simulink model "sampled_data_system"  (R2021b)
settings: Solver=ode45  StartTime=0.0  StopTime=tfinal  FixedStep=T  MaxStep=0.01  RelTol=1e-12  AbsTol=1e-12  EnableMultiTasking=on
values from neighbouring files (symbols this model uses):
  T = ts    [run.m]
libraries: cstblocks x2
settings Model: Creator=cnielsen  LastModifiedBy=Urban Pistek
settings SolverCC: AutoScaleAbsTol=off  AlgebraicLoopSolver=TrustRegion
settings DataIOCC: SaveFormat=Array  SignalLoggingSaveFormat=ModelDataLogs  SaveOutput=off  SaveTime=off  ReturnWorkspaceOutputs=off  Refine=5
settings OptimizationCC: ExpressionDepthLimit=2147483647  LifeSpan=inf
settings DebuggingCC: UnderspecifiedInitializationDetection=Classic  MergeDetectMultiDrivingBlocksExec=none  SolverPrmCheckMsg=warning  FcnCallInpInsideContextMsg=warning  StateNameClashWarn=warning  SFUnexpectedBacktrackingDiag=warning  SFNoUnconditionalDefaultTransitionDiag=warning  SFExecutionAtInitializationDiag=none  SFMachineParentedDataDiag=warning  ArithmeticOperatorsInVariantConditions=warning
settings HardwareCC: ProdBitPerPointer=32  ProdBitPerSizeT=32  ProdBitPerPtrDiffT=32  ProdLargestAtomicFloat=None  ProdIntDivRoundTo=Undefined  ProdEndianess=Unspecified  ProdWordSize=32  ProdHWDeviceType=32-bit Generic
settings ModelReferenceCC: PropagateSignalLabelsOutOfModel=off
settings SFSimCC: SimUseLocalCustomCode=off  CustomCodeUndefinedFunction=UseInterfaceOnly
settings RTWCC: RTWUseLocalCustomCode=off
settings CodeAppCC: StateflowObjectComments=on
settings GRTTargetCC: TargetLangStandard=C89/C90 (ANSI)  CombineOutputUpdateFcns=off  GRTInterface=on
settings ConfigComp: CovMetricSettings=dw  CovSaveCumulativeToWorkspaceVar=on  CovSaveSingleToWorkspaceVar=on  CovExternalEMLEnable=off

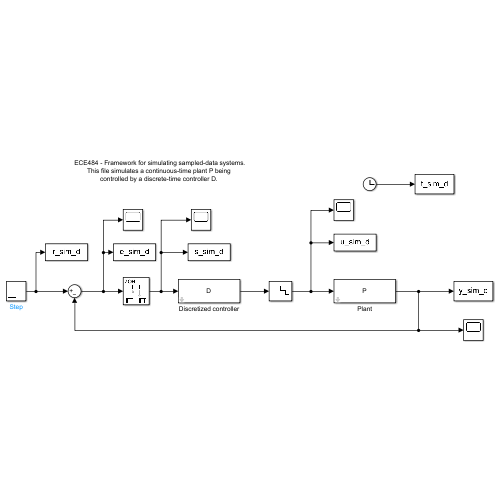
[thumbnail: Simulink's stored preview of the top-level diagram]
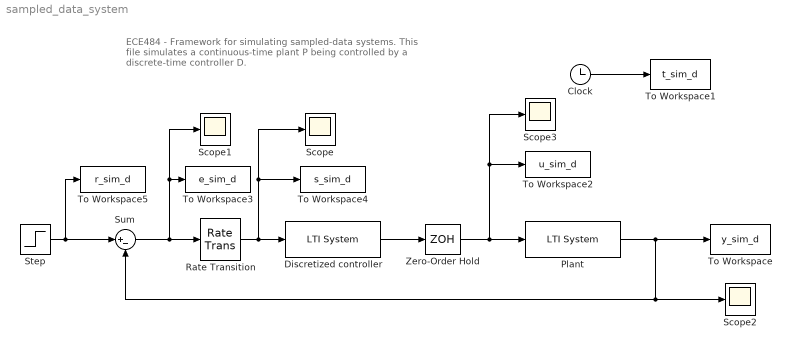
== system sampled_data_system ==
  note: ECE484 - Framework for simulating sampled-data systems.
      | This file simulates a continuous-time plant P being
      | controlled by a discrete-time controller D.
  Clock : Clock
  Discretized controller : cstblocks/LTI System  sys=D  IC=[]
  Plant : cstblocks/LTI System  sys=P  IC=[]
  Rate Transition : RateTransition  OutPortSampleTime=T
  Scope{,1..3} (4 alike) : Scope
  Step : Step  Time=0
  Sum : Sum  Inputs=|+-
  To Workspace : ToWorkspace  VariableName=y_sim_d  SampleTime=-1
  To Workspace1 : ToWorkspace  VariableName=t_sim_d  SampleTime=-1
  To Workspace2 : ToWorkspace  VariableName=u_sim_d
  To Workspace3 : ToWorkspace  VariableName=e_sim_d
  To Workspace4 : ToWorkspace  VariableName=s_sim_d
  To Workspace5 : ToWorkspace  VariableName=r_sim_d
  Zero-Order Hold : ZeroOrderHold  SampleTime=T
  wires:
  Clock/1 -> To Workspace1/1
  Discretized controller/1 -> Zero-Order Hold/1
  Step/1 -> To Workspace5/1, Sum/1
  Plant/1 -> To Workspace/1, Sum/2, Scope2/1
  Sum/1 -> Rate Transition/1, To Workspace3/1, Scope1/1
  Zero-Order Hold/1 -> Plant/1, To Workspace2/1, Scope3/1
  Rate Transition/1 -> Discretized controller/1, To Workspace4/1, Scope/1
